simulink model "flightSimulation"  (R2021b)
settings: Solver=FixedStepAuto  StartTime=0  StopTime=end_time  FixedStep=0.005  RelTol=1e-3  EnableMultiTasking=on
undefined symbols (not defined in the file or in its folder): B, builder_switch, Earth, filter_switch, ft, initEuler, initPosLLA, inv_method, m, mass, s, sigbuilder_block, sw_turb, Ts, umax, umin, Vehicle, WGS84
libraries: slpidlib x8, dspsrcs4 x6, aerolibconvert2 x4, dspswit3 x3, aerolibanimutils x2, aerolibfltsims x2, shared6dof x1, aerolibtransform2 x1, qcatlib x1, aerolibwind2 x1, aerolibgravity2 x1, dspstat3 x1
(part 1 of 3)
settings Model: Creator=The MathWorks, Inc.  LastModifiedBy=mch
settings SolverCC: AlgebraicLoopSolver=LineSearch  AutoInsertRateTranBlk=on
settings DataIOCC: LimitDataPoints=on  SaveFormat=Array  SaveOutput=off  DSMLogging=off  SaveTime=off  ReturnWorkspaceOutputs=off
settings OptimizationCC: BlockReduction=off  BufferReuse=off  LifeSpan=inf
settings DebuggingCC: AlgebraicLoopMsg=none  UnderspecifiedInitializationDetection=Classic  MergeDetectMultiDrivingBlocksExec=none  MultiTaskCondExecSysMsg=none  UnconnectedInputMsg=none  UnconnectedOutputMsg=none  UnconnectedLineMsg=none  AllowSymbolicDim=off  SFUnexpectedBacktrackingDiag=warning  SFNoUnconditionalDefaultTransitionDiag=warning  SFExecutionAtInitializationDiag=none  SFMachineParentedDataDiag=warning  ArithmeticOperatorsInVariantConditions=warning
settings HardwareCC: ProdBitPerPointer=32  ProdBitPerSizeT=32  ProdBitPerPtrDiffT=32  ProdLargestAtomicFloat=None  ProdIntDivRoundTo=Undefined  ProdEndianess=Unspecified  ProdWordSize=32  ProdHWDeviceType=32-bit Generic
settings ModelReferenceCC: PropagateSignalLabelsOutOfModel=off
settings SFSimCC: SimUseLocalCustomCode=off  CustomCodeUndefinedFunction=UseInterfaceOnly
settings RTWCC: RTWUseLocalCustomCode=off
settings CodeAppCC: StateflowObjectComments=on
settings GRTTargetCC: TargetLangStandard=C89/C90 (ANSI)
settings ConfigComp: CovMetricSettings=dw  CovSaveCumulativeToWorkspaceVar=on  CovSaveSingleToWorkspaceVar=on  CovExternalEMLEnable=off  CovSFcnEnable=off

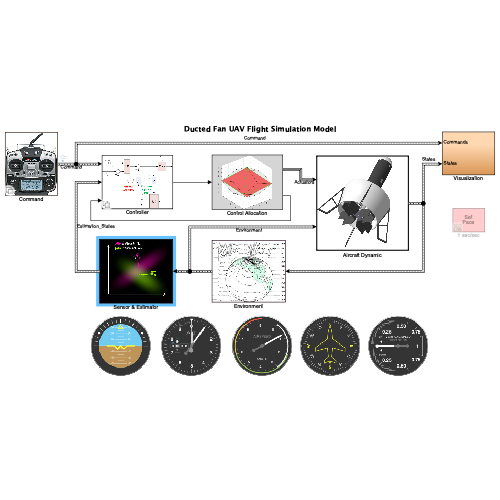
[thumbnail: Simulink's stored preview of the top-level diagram]
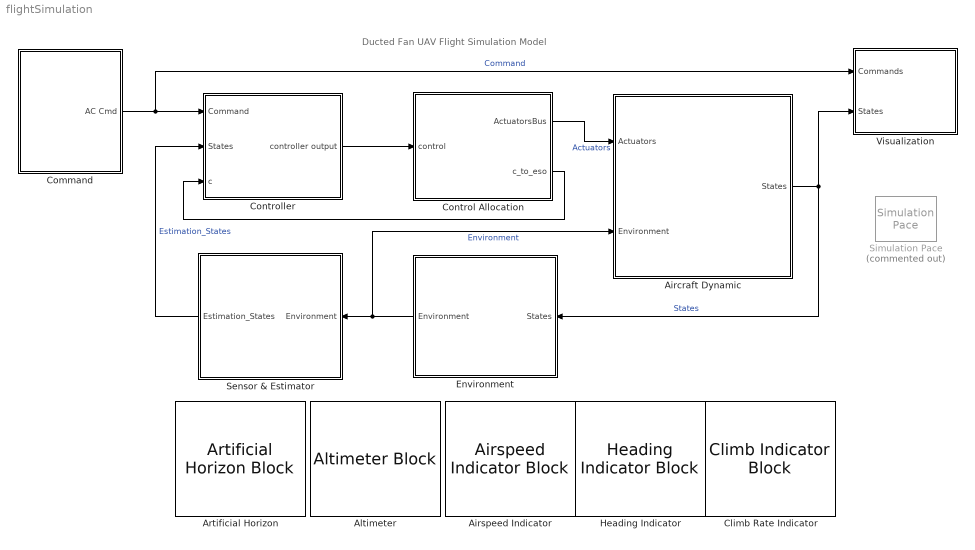
== system flightSimulation ==
  note: Ducted Fan UAV Flight Simulation Model
  Aircraft Dynamic : Subsystem  TreatAsAtomicUnit=on
      mask init:
      | vehicleNonlinearVars;
      settings: MinAlgLoopOccurrences=on
      mask Display: image('DuctedFanUAV.JPG');
  Airspeed Indicator : AirspeedIndicatorBlock  LabelPosition=Hide  ScaleMin=0  ScaleMax=9
  Altimeter : AltimeterBlock  LabelPosition=Hide
  Artificial Horizon : ArtificialHorizonBlock  LabelPosition=Hide
  Climb Rate Indicator : ClimbIndicatorBlock  LabelPosition=Hide  ScaleMax=1000
  Command : Subsystem  Variant=on
      mask Display: image('61gyiDMUFkL._AC_SX522_.jpg');
  Control Allocation : Subsystem
      mask Display: image('AMS.png');
  Controller : Subsystem  Variant=on  VariantControl=Variant1
  Environment : Subsystem
      mask Display: image('Magnetic_Storm_Oct_2003.jpg');
  Heading Indicator : HeadingIndicatorBlock  LabelPosition=Hide
  Sensor & Estimator : Subsystem
      mask Display: image('estimator.jpg');
  Simulation Pace : aerolibanimutils/Simulation Pace  Commented=on  SimulationPace=1  SleepMode=MATLAB Thread  OutputPaceError=off  SampleTime=Ts
      settings: AttributesFormatString=%<SimulationPace> sec/sec
  Visualization : Subsystem
  wires:
  Aircraft Dynamic/1(States) -> Environment/1(States), Visualization/2(States)  "States"
  Environment/1(Environment) -> Aircraft Dynamic/2(Environment), Sensor & Estimator/1(Environment)  "Environment"
  Command/1(AC Cmd) -> Visualization/1(Commands), Controller/1("Command ")  "Command"
  Control Allocation/1(ActuatorsBus) -> Aircraft Dynamic/1(Actuators)  "Actuators"
  Sensor & Estimator/1(Estimation_States) -> Controller/2(States)  "Estimation_States"
  Controller/1(controller output) -> Control Allocation/1(control)
  Control Allocation/2(c_to_eso) -> Controller/3(c)

== system flightSimulation/Aircraft Dynamic ==
  note: Plant
  note: A_be: the accelerations in body-fixed axes with respect to inertial frame (flat Earth). A_be=R_n2b*d(V^n)/dt
      | A_bb: the accelerations in body-fixed axes with respect to body frame. A_bb=d(V^b)/dt
  Actuators : Inport  OutDataTypeStr=Bus: ActuatorsBus
  Environment : Inport  Port=2  OutDataTypeStr=Bus: EnvironmentBus
  6DOF (Quaternion) : shared6dof/6DOF (Euler Angles)  units=Metric (MKS)  mtype=Fixed  rep=Euler Angles  xme_0=initPosNED  Vm_0=initVb  eul_0=initEuler  pm_0=initAngRates  mass_0=mass  mass_e=0.5  mass_f=2.0  inertia=inertia  inertia_e=eye(3)  inertia_f=2*eye(3)  k_quat=Vehicle.Nonlinear.Nonlinear.SixDOF.quatGain  vre_flag=on  abi_flag=on  aMode=aMode  xme_statename=''  Vm_statename=''  eul_statename=''  quat_statename=''  pm_statename=''  mass_statename=''
      settings: SourceProductBaseCode=AE,PW,DR,MT,UV,VE
  Bus setup : Subsystem
  Calculation force : Subsystem
  Calculation torque : Subsystem
  Position on Earth : Subsystem  Priority=1  TreatAsAtomicUnit=on
  Terminator : Terminator
  States : Outport  VectorParamsAs1DForOutWhenUnconnected=off
  wires:
  Actuators/1 -> Calculation torque/1(ActuatorsBus), Calculation force/1(ActuatorsBus)  "ActuatorsBus"
  Environment/1 -> Calculation force/2(EnvironmentBus), Calculation torque/2(EnvironmentBus)  "Environment"
  6DOF (Quaternion)/9 -> Bus setup/9(Accel_b)
  6DOF (Quaternion)/8 -> Terminator/1
  6DOF (Quaternion)/3 -> Bus setup/4(Euler)
  6DOF (Quaternion)/6 -> Bus setup/7(Omega_b)
  Calculation torque/1(M^b) -> 6DOF (Quaternion)/2
  Calculation force/1(F^b) -> 6DOF (Quaternion)/1
  Bus setup/1(States) -> States/1  "StatesBus"
  6DOF (Quaternion)/4 -> Bus setup/5(DCM_be)  "Rn2b"
  6DOF (Quaternion)/7 -> Bus setup/8(dOmega_b)
  6DOF (Quaternion)/5 -> Bus setup/6(V_b)
  6DOF (Quaternion)/2 -> Position on Earth/1(Xe), Bus setup/3(X_ned)
  6DOF (Quaternion)/1 -> Bus setup/2(V_ned)
  Position on Earth/1(LLA) -> Bus setup/1(LLA)

== system flightSimulation/Command ==
  note: VSS_COMMAND = 0 will select Signal Builder
      | VSS_COMMAND =1 will select Joystick + Signal Builder
      | VSS_COMMAND = 2 will select pre-saved data from .mat file
      | VSS_COMMAND = 3 will select user
  Data : Subsystem  VariantControl=VSS_COMMAND_PRESAVED
  Joystick : Subsystem  VariantControl=VSS_COMMAND_JOYSTICK
  Signal Builder : Subsystem  VariantControl=VSS_COMMAND_SIGBLDR
  user : Subsystem  VariantControl=VSS_COMMAND_user
  AC Cmd : Outport  OutDataTypeStr=Bus: CommandBus  VectorParamsAs1DForOutWhenUnconnected=off

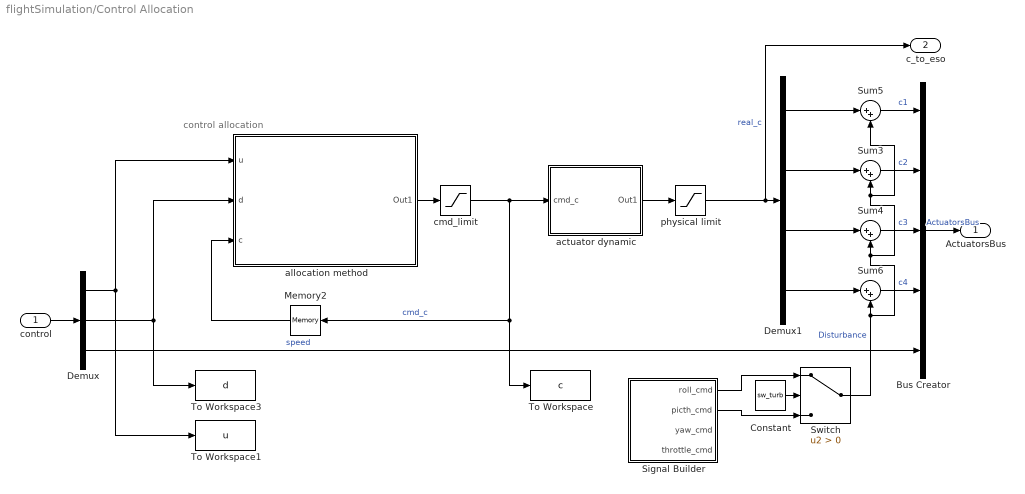
== system flightSimulation/Control Allocation ==
  note: control allocation
  control : Inport
  Bus Creator : BusCreator  Inputs=5  OutDataTypeStr=Bus: ActuatorsBus
  Constant : Constant  Value=sw_turb
  Demux : Demux  Outputs=[3,3,1]
  Demux1 : Demux
  Memory2 : Memory  InitialCondition=[0;0;0;0]  InheritSampleTime=on  LinearizeAsDelay=on
  Signal Builder : Subsystem  Tag=STV Subsys  LoadFcn=sigbuilder_block('load');  StartFcn=sigbuilder_block('start');  StopFcn=sigbuilder_block('stop');  ClipboardFcn=sigbuilder_block('clipboard');  mask(Sigbuilder block){tuvar=[0:10]}
      mask help: Simulink:masks:SigbuilderBlock_MD
      mask init:
      | if ~strcmp(get_param(bdroot(gcbh),'SimulationStatus'),'stopped') tuvar = sigbuilder_block('maskInit'); end
      settings: CopyFcn=sigbuilder_block('copy');  DeleteFcn=sigbuilder_block('delete');  ModelCloseFcn=sigbuilder_block('modelClose');  PreSaveFcn=sigbuilder_block('preSave');  PauseFcn=sigbuilder_block('pause');  ContinueFcn=sigbuilder_block('continue');  NameChangeFcn=sigbuilder_block('namechange');  OpenFcn=sigbuilder_block('open',[336 114 630 307.5 ]);  CloseFcn=sigbuilder_block('close');
      mask Display: plot(0, 0, 100, 100,[2, 2, 32, 32, 2], [68, 8, 8, 68, 68],[32, 2], [38, 38], [32, 19, 2],[53, 60, 44], [32, 17, 17, 2],[16, 16, 31, 31]);txt = getActiveGroup(gcbh);text(2, 100, txt,'verticalAlignment', 'top');
  Sum{3..6} (4 alike) : Sum  Inputs=|++
  Switch : Switch  Criteria=u2 > Threshold
  To Workspace : ToWorkspace  VariableName=c  SaveFormat=Timeseries  SampleTime=0.01
  To Workspace1 : ToWorkspace  VariableName=u  SaveFormat=Timeseries  SampleTime=0.01
  To Workspace3 : ToWorkspace  VariableName=d  SaveFormat=Timeseries  SampleTime=0.01
  actuator dynamic : Subsystem
  allocation method : Subsystem  Variant=on
  cmd_limit : Saturate  UpperLimit=umax  LowerLimit=umin
  physical limit : Saturate  UpperLimit=umax  LowerLimit=umin
  ActuatorsBus : Outport  OutDataTypeStr=Bus: ActuatorsBus  VectorParamsAs1DForOutWhenUnconnected=off
  c_to_eso : Outport  Port=2  VectorParamsAs1DForOutWhenUnconnected=off
  wires:
  Bus Creator/1 -> ActuatorsBus/1  "ActuatorsBus"
  control/1 -> Demux/1
  Demux/3 -> Bus Creator/5  "speed"
  Demux/2 -> allocation method/2(d), To Workspace3/1
  actuator dynamic/1(Out1) -> physical limit/1
  physical limit/1 -> c_to_eso/1, Demux1/1  "real_c"
  cmd_limit/1 -> actuator dynamic/1(cmd_c), To Workspace/1, Memory2/1  "cmd_c"
  Switch/1 -> Sum5/2, Sum3/2, Sum4/2, Sum6/2  "Disturbance"
  Constant/1 -> Switch/2
  Signal Builder/2(picth_cmd) -> Switch/3
  Signal Builder/1(roll_cmd) -> Switch/1
  allocation method/1(Out1) -> cmd_limit/1
  Demux1/4 -> Sum6/1
  Demux1/3 -> Sum4/1
  Demux1/2 -> Sum3/1
  Demux1/1 -> Sum5/1
  Memory2/1 -> allocation method/3(c)
  Sum6/1 -> Bus Creator/4  "c4"
  Sum4/1 -> Bus Creator/3  "c3"
  Sum3/1 -> Bus Creator/2  "c2"
  Sum5/1 -> Bus Creator/1  "c1"
  Demux/1 -> allocation method/1(u), To Workspace1/1

== system flightSimulation/Controller ==
  "Command " : Inport  OutDataTypeStr=Bus: CommandBus
  States : Inport  Port=2  OutDataTypeStr=Bus: StatesBus
  c : Inport  Port=3
  ADRC : Subsystem  VariantControl=controller==0
      mask Display: image('Block-Diagram-of-ADRC-Controller.png');
  PID : Subsystem  VariantControl=controller==1
      mask Display: image('PID_en-1024x364.jpg');
  controller output : Outport  VectorParamsAs1DForOutWhenUnconnected=off

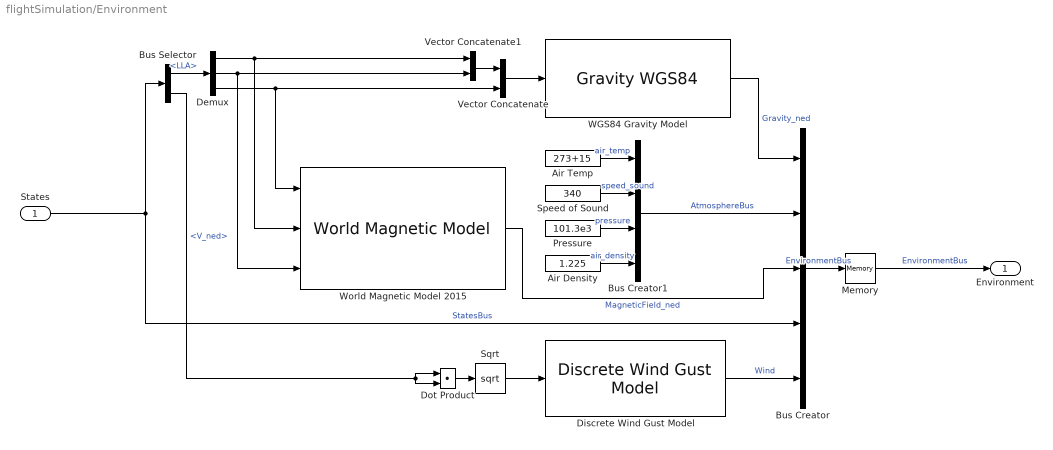
== system flightSimulation/Environment ==
  States : Inport  OutDataTypeStr=Bus: StatesBus
  Air Density : Constant  Value=1.225
  Air Temp : Constant  Value=273+15
  Bus Creator : BusCreator  Inputs=5  OutDataTypeStr=Bus: EnvironmentBus  NonVirtualBus=on
  Bus Creator1 : BusCreator  Inputs=4  OutDataTypeStr=Bus: AtmosphereBus  NonVirtualBus=on
  Bus Selector : BusSelector  OutputSignals=LLA,V_ned
  Demux : Demux  Outputs=3
  Discrete Wind Gust Model : aerolibwind2/Discrete Wind Gust Model  units=Metric (MKS)  Gx=on  Gy=on  Gz=on  t_0=120  d_m=[5 5 5]  v_m=[2 2 0]
  Dot Product : DotProduct  InputSameDT=on  OutDataTypeStr=Inherit: Inherit via internal rule
  Memory : Memory  InheritSampleTime=on
  Pressure : Constant  Value=101.3e3
  Speed of Sound : Constant  Value=340
  Sqrt : Sqrt  SaturateOnIntegerOverflow=on
  Vector Concatenate : Concatenate
  Vector Concatenate1 : Concatenate
  "WGS84 Gravity Model  " : GravityWGS84  model=WGS84 Exact  no_centrifugal=off  action=None
  World Magnetic Model 2015 : aerolibgravity2/World Magnetic Model  model=WMM2015 V2 (2015-2020)  customFile='WMM2020.COF'  units=Metric (MKS)  time_in=off  month=January  day=1  year=2015  action=Error  h_out=off  dec_out=off  inc_out=off  ti_out=off
      settings: SourceProductBaseCode=AE
  Environment : Outport  OutDataTypeStr=Bus: EnvironmentBus  VectorParamsAs1DForOutWhenUnconnected=off
  wires:
  Vector Concatenate1/1 -> Vector Concatenate/1
  States/1 -> Bus Selector/1, Bus Creator/4  "StatesBus"
  World Magnetic Model 2015/1 -> Bus Creator/3  "MagneticField_ned"
  Bus Selector/1 -> Demux/1  "<LLA>"
  Discrete Wind Gust Model/1 -> Bus Creator/5  "Wind"
  Pressure/1 -> Bus Creator1/3  "pressure"
  Air Density/1 -> Bus Creator1/4  "air_density"
  Bus Creator1/1 -> Bus Creator/2  "AtmosphereBus"
  Speed of Sound/1 -> Bus Creator1/2  "speed_sound"
  Air Temp/1 -> Bus Creator1/1  "air_temp"
  "WGS84 Gravity Model  "/1 -> Bus Creator/1  "Gravity_ned"
  Bus Creator/1 -> Memory/1  "EnvironmentBus"
  Vector Concatenate/1 -> "WGS84 Gravity Model  "/1
  Demux/1 -> World Magnetic Model 2015/2, Vector Concatenate1/1
  Demux/2 -> World Magnetic Model 2015/3, Vector Concatenate1/2
  Demux/3 -> World Magnetic Model 2015/1, Vector Concatenate/2
  Bus Selector/2 -> Dot Product/1, Dot Product/2  "<V_ned>"
  Dot Product/1 -> Sqrt/1
  Sqrt/1 -> Discrete Wind Gust Model/1
  Memory/1 -> Environment/1  "EnvironmentBus"

== system flightSimulation/Sensor & Estimator ==
  Environment : Inport  OutDataTypeStr=Bus: EnvironmentBus
  Bus Creator5 : BusCreator  Inputs=9  OutDataTypeStr=Bus: StatesBus  NonVirtualBus=on
  Bus Selector : BusSelector  OutputSignals=StatesBus,MagneticField_ned,Gravity_ned
  Bus Selector1 : BusSelector  OutputSignals=V_body,Omega_body,Euler,Accel_body,dOmega_body,V_ned,X_ned,LLA,DCM_be
  Filter : Subsystem
  Rate Transition2 : RateTransition  OutPortSampleTime=0.01
  Sensor : Subsystem
      mask Display: image('imu_mems.jpg');
  Estimation_States : Outport  OutDataTypeStr=Bus: StatesBus  VectorParamsAs1DForOutWhenUnconnected=off
  wires:
  Rate Transition2/1 -> Estimation_States/1
  Bus Creator5/1 -> Rate Transition2/1
  Environment/1 -> Bus Selector/1
  Bus Selector/1 -> Bus Selector1/1  "<StatesBus>"
  Bus Selector1/1 -> Bus Creator5/1  "<V_body>"
  Bus Selector1/5 -> Bus Creator5/5, Sensor/3(<dOmega_body>)  "<dOmega_body>"
  Bus Selector1/4 -> Bus Creator5/4, Sensor/2(<Accel_body>)  "<Accel_body>"
  Bus Selector1/8 -> Bus Creator5/8  "<LLA>"
  Bus Selector1/2 -> Sensor/1(<Omega_body>), Filter/1(omega)  "<Omega_body>"
  Bus Selector1/6 -> Bus Creator5/6, Sensor/5(<V_ned>)  "<V_ned>"
  Bus Selector1/7 -> Bus Creator5/7  "<X_ned>"
  Bus Selector1/3 -> Filter/2(euler)  "<Euler>"
  Bus Selector1/9 -> Bus Creator5/9, Sensor/7(<DCM_be>)  "<DCM_be>"
  Bus Selector/2 -> Sensor/4(<MagneticField_ned>)  "<MagneticField_ned>"
  Bus Selector/3 -> Sensor/6(<Gravity_ned>)  "<Gravity_ned>"
  Sensor/1(Out1) -> Filter/3(sensor)
  Filter/2(Euler) -> Bus Creator5/3  "Euler"
  Filter/1(Omega_body) -> Bus Creator5/2  "Omega_body"

== system flightSimulation/Visualization ==
  Commands : Inport
  States : Inport  Port=2
  Extract Flight Instruments : Subsystem
  Visualization : Subsystem  Variant=on
  wires:
  Commands/1 -> Visualization/2(Commands)
  States/1 -> Visualization/1(States), Extract Flight Instruments/1(States)

== system flightSimulation/Aircraft Dynamic/Bus setup ==
  LLA : Inport  PortDimensions=3
  V_ned : Inport  Port=2  PortDimensions=3
  X_ned : Inport  Port=3  PortDimensions=3
  Euler : Inport  Port=4  PortDimensions=3
  DCM_be : Inport  Port=5  PortDimensions=[3 3]
  V_b : Inport  Port=6  PortDimensions=3
  Omega_b : Inport  Port=7  PortDimensions=3
  dOmega_b : Inport  Port=8  PortDimensions=3
  Accel_b : Inport  Port=9  PortDimensions=3
  Bus Creator5 : BusCreator  Inputs=9  OutDataTypeStr=Bus: StatesBus  NonVirtualBus=on
  States : Outport  VectorParamsAs1DForOutWhenUnconnected=off
  wires:
  Bus Creator5/1 -> States/1
  V_b/1 -> Bus Creator5/1  "V_body"
  Omega_b/1 -> Bus Creator5/2  "Omega_body"
  Euler/1 -> Bus Creator5/3  "Euler"
  X_ned/1 -> Bus Creator5/7  "X_ned"
  Accel_b/1 -> Bus Creator5/4  "Accel_body"
  LLA/1 -> Bus Creator5/8  "LLA"
  dOmega_b/1 -> Bus Creator5/5  "dOmega_body"
  DCM_be/1 -> Bus Creator5/9  "DCM_be"
  V_ned/1 -> Bus Creator5/6  "V_ned"

== system flightSimulation/Aircraft Dynamic/Calculation force ==
  ActuatorsBus : Inport
  EnvironmentBus : Inport  Port=2
  Bus Selector : BusSelector  OutputSignals=speed,c1,c2,c3,c4
  Bus Selector1 : BusSelector  OutputSignals=StatesBus.V_body,Wind,Gravity_ned,StatesBus.DCM_be
  Demux : Demux  Outputs=3
  Demux1 : Demux  Outputs=3
  Mux1 : Mux  Inputs=11
  S-Function : S-Function  FunctionName=s_Force  SFunctionDeploymentMode=off  EnableBusSupport=off
  Subsystem1 : Subsystem
  F^b : Outport  VectorParamsAs1DForOutWhenUnconnected=off
  wires:
  ActuatorsBus/1 -> Bus Selector/1
  Demux/1 -> Mux1/6
  Demux/2 -> Mux1/7
  Mux1/1 -> S-Function/1
  Bus Selector/3 -> Mux1/3  "<c2>"
  Bus Selector1/4 -> Subsystem1/3(Rn2b)  "<DCM_be>"
  Demux1/1 -> Mux1/9
  Demux1/3 -> Mux1/11
  Demux1/2 -> Mux1/10
  Bus Selector/5 -> Mux1/5  "<c4>"
  EnvironmentBus/1 -> Bus Selector1/1
  Bus Selector/1 -> Mux1/1  "<speed>"
  Bus Selector/4 -> Mux1/4  "<c3>"
  Demux/3 -> Mux1/8
  Bus Selector1/2 -> Demux1/1  "<Wind>"
  Bus Selector1/1 -> Demux/1  "<V_body>"
  Bus Selector/2 -> Mux1/2  "<c1>"
  Bus Selector1/3 -> Subsystem1/2(g_ned)  "<Gravity_ned>"
  Subsystem1/1(F^b) -> F^b/1
  S-Function/1 -> Subsystem1/1(F)

== system flightSimulation/Aircraft Dynamic/Calculation torque ==
  ActuatorsBus : Inport  OutDataTypeStr=Bus: ActuatorsBus
  EnvironmentBus : Inport  Port=2  OutDataTypeStr=Bus: EnvironmentBus
  Bus Selector1 : BusSelector  OutputSignals=StatesBus.V_body,Wind,StatesBus.Omega_body
  Bus Selector2 : BusSelector  OutputSignals=c1,c2,c3,c4,speed
  Demux : Demux  Outputs=3
  Demux1 : Demux  Outputs=3
  Demux2 : Demux  Outputs=3
  M : S-Function  FunctionName=s_Torque  SFunctionDeploymentMode=off  EnableBusSupport=off
  Mux2 : Mux  Inputs=14
  M^b : Outport  VectorParamsAs1DForOutWhenUnconnected=off
  wires:
  Demux1/3 -> Mux2/11
  Mux2/1 -> M/1
  Demux1/2 -> Mux2/10
  Demux/3 -> Mux2/8
  Bus Selector2/3 -> Mux2/3  "<c3>"
  Demux/1 -> Mux2/6
  Bus Selector2/5 -> Mux2/5  "<speed>"
  Demux1/1 -> Mux2/9
  Bus Selector2/4 -> Mux2/4  "<c4>"
  Demux/2 -> Mux2/7
  Demux2/2 -> Mux2/13
  ActuatorsBus/1 -> Bus Selector2/1  "ActuatorsBus"
  EnvironmentBus/1 -> Bus Selector1/1  "EnvironmentBus"
  Bus Selector2/1 -> Mux2/1  "<c1>"
  Bus Selector2/2 -> Mux2/2  "<c2>"
  Bus Selector1/1 -> Demux/1  "<V_body>"
  Bus Selector1/2 -> Demux1/1  "<Wind>"
  Bus Selector1/3 -> Demux2/1  "<Omega_body>"
  Demux2/1 -> Mux2/12
  Demux2/3 -> Mux2/14
  M/1 -> M^b/1

== system flightSimulation/Aircraft Dynamic/Position on Earth ==
  Xe : Inport
  Flat Earth to LLA : aerolibtransform2/Flat Earth to LLA  units=Metric (MKS)  ptype=Earth (WGS84)  F=1/298.257223563  R=6378137  refPosPort=off  LL0=initPosLLA(1:2)  psi=Vehicle.Nonlinear.Nonlinear.PositionOnEarth.FlatEarthToLLA.xAxis
  Mux : Mux  Inputs=2
  href : Constant  Value=Vehicle.Nonlinear.Nonlinear.PositionOnEarth.href
  LLA : Outport  VectorParamsAs1DForOutWhenUnconnected=off
  wires:
  Mux/1 -> LLA/1
  Xe/1 -> Flat Earth to LLA/1
  Flat Earth to LLA/1 -> Mux/1
  Flat Earth to LLA/2 -> Mux/2
  href/1 -> Flat Earth to LLA/2

== system flightSimulation/Command/Data ==
  Bus Creator : BusCreator  Inputs=4  OutDataTypeStr=Bus: CommandBus  NonVirtualBus=on
  From Workspace : FromWorkspace  VariableName=cmdroll
  From Workspace1 : FromWorkspace  VariableName=cmdpitch
  From Workspace2 : FromWorkspace  VariableName=cmdyaw
  From Workspace3 : FromWorkspace  VariableName=cmdh
  AC Cmd : Outport  OutDataTypeStr=Bus: CommandBus  VectorParamsAs1DForOutWhenUnconnected=off
  wires:
  Bus Creator/1 -> AC Cmd/1
  From Workspace1/1 -> Bus Creator/2  "pitch_cmd"
  From Workspace2/1 -> Bus Creator/3  "yaw_cmd"
  From Workspace3/1 -> Bus Creator/4  "throttle_cmd"
  From Workspace/1 -> Bus Creator/1  "roll_cmd"

== system flightSimulation/Command/Joystick ==
  Bus Creator : BusCreator  Inputs=4  OutDataTypeStr=Bus: CommandBus  NonVirtualBus=on
  Pilot Joystick : aerolibanimutils/Pilot Joystick  JoystickID=Joystick1  OutputConfiguration=FourAxis  SampleTime=Ts
  AC Cmd : Outport  OutDataTypeStr=Bus: CommandBus  VectorParamsAs1DForOutWhenUnconnected=off
  wires:
  Pilot Joystick/4 -> Bus Creator/4  "throttle_cmd"
  Pilot Joystick/3 -> Bus Creator/3  "yaw_cmd"
  Pilot Joystick/2 -> Bus Creator/2  "pitch_cmd"
  Pilot Joystick/1 -> Bus Creator/1  "roll_cmd"
  Bus Creator/1 -> AC Cmd/1

== system flightSimulation/Command/Signal Builder ==
  Bus Creator : BusCreator  Inputs=4  OutDataTypeStr=Bus: CommandBus  NonVirtualBus=on
  Bus Creator1 : BusCreator  Inputs=4  OutDataTypeStr=Bus: CommandBus  NonVirtualBus=on
  Constant : Constant  Value=builder_switch
  Signal Builder_Disturbance : Subsystem  Tag=STV Subsys  LoadFcn=sigbuilder_block('load');  StartFcn=sigbuilder_block('start');  StopFcn=sigbuilder_block('stop');  ClipboardFcn=sigbuilder_block('clipboard');  mask(Sigbuilder block){tuvar=[0:10]}
      mask help: Simulink:masks:SigbuilderBlock_MD
      mask init:
      | if ~strcmp(get_param(bdroot(gcbh),'SimulationStatus'),'stopped') tuvar = sigbuilder_block('maskInit'); end
      settings: CopyFcn=sigbuilder_block('copy');  DeleteFcn=sigbuilder_block('delete');  ModelCloseFcn=sigbuilder_block('modelClose');  PreSaveFcn=sigbuilder_block('preSave');  PauseFcn=sigbuilder_block('pause');  ContinueFcn=sigbuilder_block('continue');  NameChangeFcn=sigbuilder_block('namechange');  OpenFcn=sigbuilder_block('open',[3 6 804 505.5 ]);  CloseFcn=sigbuilder_block('close');
      mask Display: plot(0, 0, 100, 100,[2, 2, 32, 32, 2], [68, 8, 8, 68, 68],[32, 2], [38, 38], [32, 19, 2],[53, 60, 44], [32, 17, 17, 2],[16, 16, 31, 31]);txt = getActiveGroup(gcbh);text(2, 100, txt,'verticalAlignment', 'top');
  Signal Builder_noDisturbance : Subsystem  Tag=STV Subsys  LoadFcn=sigbuilder_block('load');  StartFcn=sigbuilder_block('start');  StopFcn=sigbuilder_block('stop');  ClipboardFcn=sigbuilder_block('clipboard');  mask(Sigbuilder block){tuvar=[0:10]}
      mask help: Simulink:masks:SigbuilderBlock_MD
      mask init:
      | if ~strcmp(get_param(bdroot(gcbh),'SimulationStatus'),'stopped') tuvar = sigbuilder_block('maskInit'); end
      settings: CopyFcn=sigbuilder_block('copy');  DeleteFcn=sigbuilder_block('delete');  ModelCloseFcn=sigbuilder_block('modelClose');  PreSaveFcn=sigbuilder_block('preSave');  PauseFcn=sigbuilder_block('pause');  ContinueFcn=sigbuilder_block('continue');  NameChangeFcn=sigbuilder_block('namechange');  OpenFcn=sigbuilder_block('open',[6 30 1012.5 446.25 ]);  CloseFcn=sigbuilder_block('close');
      mask Display: plot(0, 0, 100, 100,[2, 2, 32, 32, 2], [68, 8, 8, 68, 68],[32, 2], [38, 38], [32, 19, 2],[53, 60, 44], [32, 17, 17, 2],[16, 16, 31, 31]);txt = getActiveGroup(gcbh);text(2, 100, txt,'verticalAlignment', 'top');
  Switch : Switch  Criteria=u2 > Threshold
  AC Cmd : Outport  OutDataTypeStr=Bus: CommandBus  VectorParamsAs1DForOutWhenUnconnected=off
  wires:
  Bus Creator/1 -> Switch/1
  Signal Builder_Disturbance/4(throttle_cmd) -> Bus Creator/4  "throttle_cmd"
  Signal Builder_Disturbance/2(picth_cmd) -> Bus Creator/2  "pitch_cmd"
  Signal Builder_Disturbance/3(yaw_cmd) -> Bus Creator/3  "yaw_cmd"
  Signal Builder_Disturbance/1(roll_cmd) -> Bus Creator/1  "roll_cmd"
  Signal Builder_noDisturbance/1(roll_cmd) -> Bus Creator1/1
  Signal Builder_noDisturbance/2(picth_cmd) -> Bus Creator1/2
  Signal Builder_noDisturbance/3(yaw_cmd) -> Bus Creator1/3
  Signal Builder_noDisturbance/4(throttle_cmd) -> Bus Creator1/4
  Bus Creator1/1 -> Switch/3
  Switch/1 -> AC Cmd/1
  Constant/1 -> Switch/2

== system flightSimulation/Command/user ==
  Bus Creator : BusCreator  Inputs=4  OutDataTypeStr=Bus: CommandBus  NonVirtualBus=on
  Signal Builder : Subsystem  Tag=STV Subsys  LoadFcn=sigbuilder_block('load');  StartFcn=sigbuilder_block('start');  StopFcn=sigbuilder_block('stop');  ClipboardFcn=sigbuilder_block('clipboard');  mask(Sigbuilder block){tuvar=[0:10]}
      mask help: Simulink:masks:SigbuilderBlock_MD
      mask init:
      | if ~strcmp(get_param(bdroot(gcbh),'SimulationStatus'),'stopped') tuvar = sigbuilder_block('maskInit'); end
      settings: CopyFcn=sigbuilder_block('copy');  DeleteFcn=sigbuilder_block('delete');  ModelCloseFcn=sigbuilder_block('modelClose');  PreSaveFcn=sigbuilder_block('preSave');  PauseFcn=sigbuilder_block('pause');  ContinueFcn=sigbuilder_block('continue');  NameChangeFcn=sigbuilder_block('namechange');  OpenFcn=sigbuilder_block('open',[6 30 1012.5 446.25 ]);  CloseFcn=sigbuilder_block('close');
      mask Display: plot(0, 0, 100, 100,[2, 2, 32, 32, 2], [68, 8, 8, 68, 68],[32, 2], [38, 38], [32, 19, 2],[53, 60, 44], [32, 17, 17, 2],[16, 16, 31, 31]);txt = getActiveGroup(gcbh);text(2, 100, txt,'verticalAlignment', 'top');
  AC Cmd : Outport  OutDataTypeStr=Bus: CommandBus  VectorParamsAs1DForOutWhenUnconnected=off
  wires:
  Bus Creator/1 -> AC Cmd/1
  Signal Builder/1(roll_cmd) -> Bus Creator/1  "roll_cmd"
  Signal Builder/2(picth_cmd) -> Bus Creator/2  "pitch_cmd"
  Signal Builder/3(yaw_cmd) -> Bus Creator/3  "yaw_cmd"
  Signal Builder/4(throttle_cmd) -> Bus Creator/4  "throttle_cmd"

== system flightSimulation/Control Allocation/Signal Builder ==
  Demux : Demux  Tag=STV Demux
      settings: DisplayOption=none
  FromWs : FromWorkspace  Tag=STV FromWs  VariableName=tuvar
      SigBuilderData=|
      | common.afterFinalStr = 'Extrapolate'
      | common.sampleTime = 0
      | dataSet.timeRange = [0 100]
      | dataSet.name = 'Group 1'
      | sbobj.Groups.Name = 'Group 1'
      | sbobj.Groups.Signals(1).Name = 'roll_cmd'
      | sbobj.Groups.Signals(1).XData = [0 0.5 5 100]
      | sbobj.Groups.Signals(1).YData = [0 0 -0.157079632679 -0.157079632679]
      | sbobj.Groups.Signals(2).Name = 'picth_cmd'
      | sbobj.Groups.Signals(2).XData = [0 30 100]
      | sbobj.Groups.Signals(2).YData = [0 0 0]
      | sbobj.Groups.Signals(3).Name = 'yaw_cmd'
      | sbobj.Groups.Signals(3).XData = [0 30 30 100]
      | sbobj.Groups.Signals(3).YData = [0.0779 0.0779 0.2 0.2]
      | sbobj.Groups.Signals(4).Name = 'throttle_cmd'
      | sbobj.Groups.Signals(4).XData = [0 0.55 5 100]
      | sbobj.Groups.Signals(4).YData = [0 0 -0.17 -0.17]
      | sbobj.Groups.TimeRange = [0 100]
  roll_cmd : Outport  Tag=STV Outport  VectorParamsAs1DForOutWhenUnconnected=off
  picth_cmd : Outport  Tag=STV Outport  Port=2  VectorParamsAs1DForOutWhenUnconnected=off
  yaw_cmd : Outport  Tag=STV Outport  Port=3  VectorParamsAs1DForOutWhenUnconnected=off
  throttle_cmd : Outport  Tag=STV Outport  Port=4  VectorParamsAs1DForOutWhenUnconnected=off
  wires:
  Demux/1 -> roll_cmd/1
  FromWs/1 -> Demux/1
  Demux/2 -> picth_cmd/1
  Demux/3 -> yaw_cmd/1
  Demux/4 -> throttle_cmd/1

== system flightSimulation/Control Allocation/actuator dynamic ==
  cmd_c : Inport
  Demux3 : Demux
  Mux1 : Mux
  Rate Transition : RateTransition
  Transfer Fcnnon{1..4} (4 alike) : TransferFcn  Numerator=45  Denominator=[1 45]
  actuator dynamics compensate : Subsystem
  Out1 : Outport  VectorParamsAs1DForOutWhenUnconnected=off
  wires:
  Demux3/1 -> Transfer Fcnnon4/1
  Transfer Fcnnon3/1 -> Mux1/4  "c4"
  Demux3/2 -> Transfer Fcnnon1/1
  Demux3/3 -> Transfer Fcnnon2/1
  Transfer Fcnnon4/1 -> Mux1/1  "c1"
  Demux3/4 -> Transfer Fcnnon3/1
  Mux1/1 -> Out1/1
  Transfer Fcnnon2/1 -> Mux1/3  "c3"
  Transfer Fcnnon1/1 -> Mux1/2  "c2"
  cmd_c/1 -> Rate Transition/1
  Rate Transition/1 -> actuator dynamics compensate/1(In1)
  actuator dynamics compensate/1(Out1) -> Demux3/1

== system flightSimulation/Control Allocation/allocation method ==
  note: 0: inv
      | 1:dir
      | 2:pro
      | 3:qp
  u : Inport
  d : Inport  Port=2
  c : Inport  Port=3
  dir : Subsystem  VariantControl=allocatiom_method==1
  inv : Subsystem  VariantControl=allocatiom_method==0
  pro : Subsystem  VariantControl=allocatiom_method==2
  qp : Subsystem  VariantControl=allocatiom_method==3
  Out1 : Outport  VectorParamsAs1DForOutWhenUnconnected=off

== system flightSimulation/Controller/ADRC ==
  Command : Inport
  States : Inport  Port=2  OutDataTypeStr=Bus: StatesBus
  c : Inport  Port=3
  Bus Selector : BusSelector  OutputSignals=roll_cmd,pitch_cmd,yaw_cmd,throttle_cmd
  Bus Selector1 : BusSelector  OutputSignals=Euler,Omega_body,X_ned
  Mux : Mux  Inputs=[3,3,1]
  Rate Transition : RateTransition  OutPortSampleTime=0.01
  attitude controller : Subsystem
  high controler : Subsystem
  controller output : Outport  VectorParamsAs1DForOutWhenUnconnected=off
  wires:
  Command/1 -> Rate Transition/1
  States/1 -> Bus Selector1/1
  Bus Selector1/1 -> high controler/2(<Euler>), attitude controller/5(<Euler>)  "<Euler>"
  Bus Selector/1 -> attitude controller/1(<roll_cmd>)  "<roll_cmd>"
  Bus Selector/2 -> attitude controller/2(<pitch_cmd>)  "<pitch_cmd>"
  Bus Selector/3 -> attitude controller/3(<yaw_cmd>)  "<yaw_cmd>"
  Bus Selector1/2 -> attitude controller/6(<Omega_body>)  "<Omega_body>"
  Bus Selector/4 -> high controler/1(<throttle_cmd>)  "<throttle_cmd>"
  Bus Selector1/3 -> high controler/3(<X_ned>)  "<X_ned>"
  high controler/1(speed) -> Mux/3
  attitude controller/1(virtual control) -> Mux/1
  attitude controller/2(turb) -> Mux/2
  Mux/1 -> controller output/1
  Rate Transition/1 -> Bus Selector/1
  c/1 -> attitude controller/4(c)
